simulink library "lib_exhaust2"  (Simulink 5.0)
values from neighbouring files (symbols this model uses):
  logFlag = 1    [advSACompMaskInit.m]    (also in advSACompMaskInitR13.m)
undefined symbols (not defined in the file or in its folder): amb_tmp, cyc_mph, ex_cat_co_frac, ex_cat_ext_cp, ex_cat_ext_emisv, ex_cat_ext_init_tmp, ex_cat_ext_mass, ex_cat_ext_sarea, ex_cat_hc_frac, ex_cat_i2p_th_cond, ex_cat_i2x_emisv, ex_cat_i2x_th_cond, ex_cat_int_cp, ex_cat_int_init_tmp, ex_cat_int_mass, ex_cat_int_sarea, ex_cat_lim, ex_cat_m2i_th_cond, ex_cat_m2i_tmp, ex_cat_m2p_emisv, ex_cat_mon_cp, ex_cat_mon_init_tmp, ex_cat_mon_mass, ex_cat_mon_sarea, ex_cat_monf_sarea, ex_cat_moni_sarea, ex_cat_nox_frac, ex_cat_p2x_th_cond, ex_cat_pcm_ecp, ex_cat_pcm_mass, ex_cat_pcm_tmp, ex_cat_pipe_cp, ex_cat_pipe_emisv, ex_cat_pipe_init_tmp, ex_cat_pipe_mass, ex_cat_pipe_sarea, ex_cat_pm_frac, ex_cat_tmp_range, ex_gas_cp, ex_manif_cp, ex_manif_emisv, ex_manif_init_tmp, ex_manif_mass, ex_manif_sarea, ex_ornl_bool, fc_pwr_scale, magnitude
settings Model: LastModifiedBy=mokeefe
settings Model: ModifiedComment=|
  | mokeefe -- Thu Apr 18 08:32:39 2002 -- Version 1.56
  | saving the model:
  | o "without the model browser open"
  | o with only top-level screen visible
  | o with "fit to view" enabled
  | o with "status bar" off and "toolbar" off
  | o with "prompt to update model history with each save" on
settings Model: ModifiedHistory=|
  | mokeefe -- Thu Apr 18 08:32:39 2002 -- Version 1.56
  | saving the model:
  | o "without the model browser open"
  | o with only top-level screen visible
  | o with "fit to view" enabled
  | o with "status bar" off and "toolbar" off
  | o with "prompt to update model history with each save" on
  | 
  | mokeefe -- Thu Apr 18 08:32:39 2002 -- Version 1.56
  | saving the model:
  | o "without the model browser open"
  | o with only top-level screen visible
  | o with "fit to view" enabled
  | o with "status bar" off and "toolbar" off
  | o with "prompt to update model history with each save" on

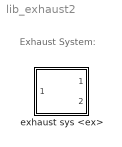
== system lib_exhaust2 ==
  note: Exhaust System:
  exhaust sys <ex> : Subsystem  TreatAsAtomicUnit=on  mask{generalName='ex', logPick=Don't Log, initFileName={}, modCell={}, imgFileName='bdi_ex.jpg', DEBUG=ON}
      mask prompts: generalName "General Name of this Component [char--evaluated]"; logPick "Log Variables to Workspace?"; initFileName "Initialization File(s) [cell array of char]"; modCell "Modification Cell [2 column cell array of param and val]"; imgFileName "Icon image file name [char--evaluated]"
      mask init:
      | % initialization via m-file script
      | advSACompMaskInitR13;
      mask StyleString: edit,popup(Don't Log|Log),edit,edit,edit,popup(ON|OFF)
      mask Display: image(imread(imgFileName))

== system lib_exhaust2/exhaust sys <ex> ==
  EO emis info : Inport
  Exhaust System Model and Interface : Subsystem
  tailpipe emis (g/s) : Outport  OutputWhenDisabled=reset  InitialOutput=0
  cat tmp (C) : Outport  Port=2  OutputWhenDisabled=reset  InitialOutput=0
  tag scope: exReqOut=global, exSensors=global
  wires:
  EO emis info/1 -> Exhaust System Model and Interface/1(EO emis info), [exReqOut]
  Exhaust System Model and Interface/1(tailpipe emis (g/s)) -> tailpipe emis (g/s)/1
  Exhaust System Model and Interface/2(cat tmp (C)) -> cat tmp (C)/1
  [exControl] -> Exhaust System Model and Interface/2(controls)
  Exhaust System Model and Interface/3(sensors) -> [exSensors]

== system lib_exhaust2/exhaust sys <ex>/Exhaust System Model and Interface ==
  note: Interface
  EO emis info : Inport
  controls : Inport  Port=2
  Bus Creator : BusCreator  Inputs=2
  Demux : Demux  Outputs=2
  Goto Tag Visibility : GotoTagVisibility  GotoTag=fc_on
  Model : Subsystem
  tailpipe emis (g/s) : Outport  OutputWhenDisabled=reset  InitialOutput=0
  cat tmp (C) : Outport  Port=2  OutputWhenDisabled=reset  InitialOutput=0
  sensors : Outport  Port=3  OutputWhenDisabled=reset  InitialOutput=0
  tag scope: fc_on=scoped
  wires:
  EO emis info/1 -> Model/1(In1)
  Model/1(tailpipe emis (g/s)) -> tailpipe emis (g/s)/1
  Model/2(cat tmp (C)) -> cat tmp (C)/1
  Bus Creator/1 -> sensors/1

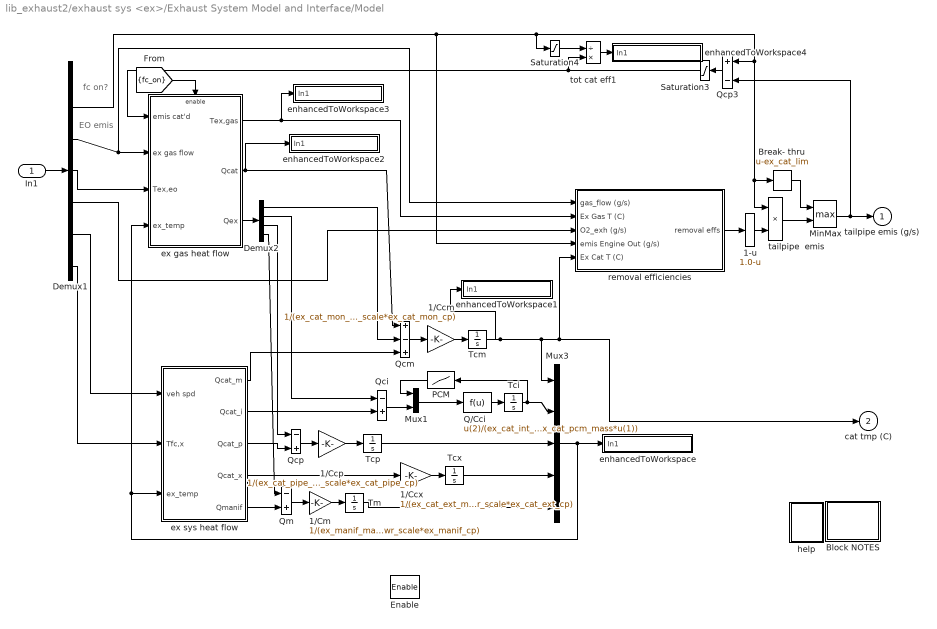
== system lib_exhaust2/exhaust sys <ex>/Exhaust System Model and Interface/Model ==
  note: fc on?
  note: EO emis
  In1 : Inport
  Enable : EnablePort  StatesWhenEnabling=reset
  1-u : MATLABFcn  MATLABFcn=1.0-u
  1/Ccm : Gain  Gain=1/(ex_cat_mon_mass*fc_pwr_scale*ex_cat_mon_cp)  SaturateOnIntegerOverflow=on
  1/Ccp : Gain  Gain=1/(ex_cat_pipe_mass*fc_pwr_scale*ex_cat_pipe_cp)  SaturateOnIntegerOverflow=on
  1/Ccx : Gain  Gain=1/(ex_cat_ext_mass*fc_pwr_scale*ex_cat_ext_cp)  SaturateOnIntegerOverflow=on
  1/Cm : Gain  Gain=1/(ex_manif_mass*fc_pwr_scale*ex_manif_cp)  SaturateOnIntegerOverflow=on
  Block NOTES : Subsystem
      mask Display: disp('Block\nNOTES')
  Break- thru : MATLABFcn  MATLABFcn=u-ex_cat_lim
  Demux1 : Demux  Outputs=[1 4 1 1 1 1 4]
  Demux2 : Demux
  MinMax : MinMax  Function=max  Inputs=2
  Mux1 : Mux  Inputs=2
  Mux3 : Mux  Inputs=5
  PCM : Lookup  Orientation=left  InputValues=ex_cat_pcm_tmp  OutputValues=ex_cat_pcm_ecp  SaturateOnIntegerOverflow=on
  Q/Cci : Fcn  Expr=u(2)/(ex_cat_int_mass*fc_pwr_scale*ex_cat_int_cp+ex_cat_pcm_mass*u(1))
  Qci : Sum  Inputs=-+  SaturateOnIntegerOverflow=on  InputSameDT=on
  Qcm : Sum  Inputs=+-+  SaturateOnIntegerOverflow=on  InputSameDT=on
  Qcp : Sum  Inputs=-+  SaturateOnIntegerOverflow=on  InputSameDT=on
  Qcp3 : Sum  Orientation=left  Inputs=+-  SaturateOnIntegerOverflow=on  InputSameDT=on
  Qm : Sum  Inputs=-+  SaturateOnIntegerOverflow=on  InputSameDT=on
  Saturation3 : Saturate  Orientation=left  UpperLimit=Inf  LowerLimit=0
  Saturation4 : Saturate  UpperLimit=Inf  LowerLimit=eps
  Tci : Integrator  InitialCondition=ex_cat_int_init_tmp
  Tcm : Integrator  InitialCondition=ex_cat_mon_init_tmp
  Tcp : Integrator  InitialCondition=ex_cat_pipe_init_tmp
  Tcx : Integrator  InitialCondition=ex_cat_ext_init_tmp
  Tm : Integrator  InitialCondition=ex_manif_init_tmp
  enhancedToWorkspace : Subsystem  TreatAsAtomicUnit=on  mask(enhancedToWorkspace){generalName=generalName, specificName=tmp, logFlag=logFlag}
      mask prompts: generalName "General Name [char-evaluated]"; specificName "Specific Name [char-literal]"; logFlag "Enable flag (1=on,0=off)"
      mask help: A wrapper for the Simulink "To Workspace" block that allows you to evaluate the name of the variable to log to workspace. This is useful to avoid the double logging errors that occur when you pull in two library models that attempt to log to the same variable.
      mask init:
      | enhancedToWsMaker
      settings: CopyFcn=breakLinkCopyFcn  ParentCloseFcn=breakLinkParCloseFcn
      mask Help:
      | <h2>Enhanced To Workspace Block</h2>
      | <h3>Parameters</h3>
      | <UL>
      | <li><b>General Name:</b> This is the more general name of the variable. Variables are saved to the workspace as <i>generalName_specificName</i>. Note that this is an evaluated variable. If you would like to type in the value directly, it must be surrounded with single quotes. Otherwise you can input the name of a variable containing a char string.</li>
      | <li><b>Specific Name:</b> This is the specific name of the variable. Note that this is input as a char literal (i.e., you don't need quotes).</li>
      | <li><b>Enable Flag:</b> This flag should have the value of 0 or 1. If 0, the variable will not be logged to the workspace. If 1, the variable will be logged. This is done so that variable logging can be turned off to improve speed.</li>
      | </ul>
      | <h3>Overview</h3>
      | <p>The enhanced to workspace block was put together to allow one to dynamically resolve variable names at run time in simulink. This is most powerful when used in conjunction with a masked subsystem to allow multiple instances of that masked subsytem to be used in the same model. The strategy is to set the generalName in the block mask which will allow the block to change the general name for all variable logging on the fly.
      | <h3>Helper Files</h3>
      | <p>Three m-files are required by the enhancedToWorkspace block. These files are located in the &lt; ADVISOR root &gt;/GUI directory :
      | <ul>
      | <li><i>enhancedToWsMaker.m</i> This file runs the mask initialization for the block</li>
      | <li><i>breakLinkCopyFcn.m</i> This file is used by the block callback when the simulink block is copied. It is necessary to break the link to the enhancedToWorkspace similar to the To Workspace block in order for it to be able to configure itself. (Try copying simulink's To Workspace block--it is impossible to make a link)</li>
      | <li><i>breakLinkParCloseFcn.m</i> This file is similar to the breakLinkCopyFcn and is used when a parent system is closed</li>
      | </ul>
      | <hr>
      | 
      | <p>Created 2003-Jan-21, Michael Patrick O'Keefe, NREL</p>
      | 
      | <!--
      | <VARDEF>
      | <H3>var_name</H3>
      | <UL>
      | <LI><B>data type</B> data type here</LI>
      | <LI><B>units</B> units here</LI>
      | <LI><B>vehicle type</B> vehicle type here</LI>
      | <LI><B>description</B> description here</LI>
      | </UL>
      | </VARDEF>
      | -->
      mask Display: disp([generalName,'_',specificName])
  enhancedToWorkspace1 : Subsystem  TreatAsAtomicUnit=on  mask(enhancedToWorkspace){generalName=generalName, specificName=cat_tmp, logFlag=logFlag}
      mask prompts: generalName "General Name [char-evaluated]"; specificName "Specific Name [char-literal]"; logFlag "Enable flag (1=on,0=off)"
      mask help: A wrapper for the Simulink "To Workspace" block that allows you to evaluate the name of the variable to log to workspace. This is useful to avoid the double logging errors that occur when you pull in two library models that attempt to log to the same variable.
      mask init:
      | enhancedToWsMaker
      settings: CopyFcn=breakLinkCopyFcn  ParentCloseFcn=breakLinkParCloseFcn
      mask Help:
      | <h2>Enhanced To Workspace Block</h2>
      | <h3>Parameters</h3>
      | <UL>
      | <li><b>General Name:</b> This is the more general name of the variable. Variables are saved to the workspace as <i>generalName_specificName</i>. Note that this is an evaluated variable. If you would like to type in the value directly, it must be surrounded with single quotes. Otherwise you can input the name of a variable containing a char string.</li>
      | <li><b>Specific Name:</b> This is the specific name of the variable. Note that this is input as a char literal (i.e., you don't need quotes).</li>
      | <li><b>Enable Flag:</b> This flag should have the value of 0 or 1. If 0, the variable will not be logged to the workspace. If 1, the variable will be logged. This is done so that variable logging can be turned off to improve speed.</li>
      | </ul>
      | <h3>Overview</h3>
      | <p>The enhanced to workspace block was put together to allow one to dynamically resolve variable names at run time in simulink. This is most powerful when used in conjunction with a masked subsystem to allow multiple instances of that masked subsytem to be used in the same model. The strategy is to set the generalName in the block mask which will allow the block to change the general name for all variable logging on the fly.
      | <h3>Helper Files</h3>
      | <p>Three m-files are required by the enhancedToWorkspace block. These files are located in the &lt; ADVISOR root &gt;/GUI directory :
      | <ul>
      | <li><i>enhancedToWsMaker.m</i> This file runs the mask initialization for the block</li>
      | <li><i>breakLinkCopyFcn.m</i> This file is used by the block callback when the simulink block is copied. It is necessary to break the link to the enhancedToWorkspace similar to the To Workspace block in order for it to be able to configure itself. (Try copying simulink's To Workspace block--it is impossible to make a link)</li>
      | <li><i>breakLinkParCloseFcn.m</i> This file is similar to the breakLinkCopyFcn and is used when a parent system is closed</li>
      | </ul>
      | <hr>
      | 
      | <p>Created 2003-Jan-21, Michael Patrick O'Keefe, NREL</p>
      | 
      | <!--
      | <VARDEF>
      | <H3>var_name</H3>
      | <UL>
      | <LI><B>data type</B> data type here</LI>
      | <LI><B>units</B> units here</LI>
      | <LI><B>vehicle type</B> vehicle type here</LI>
      | <LI><B>description</B> description here</LI>
      | </UL>
      | </VARDEF>
      | -->
      mask Display: disp([generalName,'_',specificName])
  enhancedToWorkspace2 : Subsystem  TreatAsAtomicUnit=on  mask(enhancedToWorkspace){generalName=generalName, specificName=cat_th_pwr, logFlag=logFlag}
      mask prompts: generalName "General Name [char-evaluated]"; specificName "Specific Name [char-literal]"; logFlag "Enable flag (1=on,0=off)"
      mask help: A wrapper for the Simulink "To Workspace" block that allows you to evaluate the name of the variable to log to workspace. This is useful to avoid the double logging errors that occur when you pull in two library models that attempt to log to the same variable.
      mask init:
      | enhancedToWsMaker
      settings: CopyFcn=breakLinkCopyFcn  ParentCloseFcn=breakLinkParCloseFcn
      mask Help:
      | <h2>Enhanced To Workspace Block</h2>
      | <h3>Parameters</h3>
      | <UL>
      | <li><b>General Name:</b> This is the more general name of the variable. Variables are saved to the workspace as <i>generalName_specificName</i>. Note that this is an evaluated variable. If you would like to type in the value directly, it must be surrounded with single quotes. Otherwise you can input the name of a variable containing a char string.</li>
      | <li><b>Specific Name:</b> This is the specific name of the variable. Note that this is input as a char literal (i.e., you don't need quotes).</li>
      | <li><b>Enable Flag:</b> This flag should have the value of 0 or 1. If 0, the variable will not be logged to the workspace. If 1, the variable will be logged. This is done so that variable logging can be turned off to improve speed.</li>
      | </ul>
      | <h3>Overview</h3>
      | <p>The enhanced to workspace block was put together to allow one to dynamically resolve variable names at run time in simulink. This is most powerful when used in conjunction with a masked subsystem to allow multiple instances of that masked subsytem to be used in the same model. The strategy is to set the generalName in the block mask which will allow the block to change the general name for all variable logging on the fly.
      | <h3>Helper Files</h3>
      | <p>Three m-files are required by the enhancedToWorkspace block. These files are located in the &lt; ADVISOR root &gt;/GUI directory :
      | <ul>
      | <li><i>enhancedToWsMaker.m</i> This file runs the mask initialization for the block</li>
      | <li><i>breakLinkCopyFcn.m</i> This file is used by the block callback when the simulink block is copied. It is necessary to break the link to the enhancedToWorkspace similar to the To Workspace block in order for it to be able to configure itself. (Try copying simulink's To Workspace block--it is impossible to make a link)</li>
      | <li><i>breakLinkParCloseFcn.m</i> This file is similar to the breakLinkCopyFcn and is used when a parent system is closed</li>
      | </ul>
      | <hr>
      | 
      | <p>Created 2003-Jan-21, Michael Patrick O'Keefe, NREL</p>
      | 
      | <!--
      | <VARDEF>
      | <H3>var_name</H3>
      | <UL>
      | <LI><B>data type</B> data type here</LI>
      | <LI><B>units</B> units here</LI>
      | <LI><B>vehicle type</B> vehicle type here</LI>
      | <LI><B>description</B> description here</LI>
      | </UL>
      | </VARDEF>
      | -->
      mask Display: disp([generalName,'_',specificName])
  enhancedToWorkspace3 : Subsystem  TreatAsAtomicUnit=on  mask(enhancedToWorkspace){generalName=generalName, specificName=gas_tmp, logFlag=logFlag}
      mask prompts: generalName "General Name [char-evaluated]"; specificName "Specific Name [char-literal]"; logFlag "Enable flag (1=on,0=off)"
      mask help: A wrapper for the Simulink "To Workspace" block that allows you to evaluate the name of the variable to log to workspace. This is useful to avoid the double logging errors that occur when you pull in two library models that attempt to log to the same variable.
      mask init:
      | enhancedToWsMaker
      settings: CopyFcn=breakLinkCopyFcn  ParentCloseFcn=breakLinkParCloseFcn
      mask Help:
      | <h2>Enhanced To Workspace Block</h2>
      | <h3>Parameters</h3>
      | <UL>
      | <li><b>General Name:</b> This is the more general name of the variable. Variables are saved to the workspace as <i>generalName_specificName</i>. Note that this is an evaluated variable. If you would like to type in the value directly, it must be surrounded with single quotes. Otherwise you can input the name of a variable containing a char string.</li>
      | <li><b>Specific Name:</b> This is the specific name of the variable. Note that this is input as a char literal (i.e., you don't need quotes).</li>
      | <li><b>Enable Flag:</b> This flag should have the value of 0 or 1. If 0, the variable will not be logged to the workspace. If 1, the variable will be logged. This is done so that variable logging can be turned off to improve speed.</li>
      | </ul>
      | <h3>Overview</h3>
      | <p>The enhanced to workspace block was put together to allow one to dynamically resolve variable names at run time in simulink. This is most powerful when used in conjunction with a masked subsystem to allow multiple instances of that masked subsytem to be used in the same model. The strategy is to set the generalName in the block mask which will allow the block to change the general name for all variable logging on the fly.
      | <h3>Helper Files</h3>
      | <p>Three m-files are required by the enhancedToWorkspace block. These files are located in the &lt; ADVISOR root &gt;/GUI directory :
      | <ul>
      | <li><i>enhancedToWsMaker.m</i> This file runs the mask initialization for the block</li>
      | <li><i>breakLinkCopyFcn.m</i> This file is used by the block callback when the simulink block is copied. It is necessary to break the link to the enhancedToWorkspace similar to the To Workspace block in order for it to be able to configure itself. (Try copying simulink's To Workspace block--it is impossible to make a link)</li>
      | <li><i>breakLinkParCloseFcn.m</i> This file is similar to the breakLinkCopyFcn and is used when a parent system is closed</li>
      | </ul>
      | <hr>
      | 
      | <p>Created 2003-Jan-21, Michael Patrick O'Keefe, NREL</p>
      | 
      | <!--
      | <VARDEF>
      | <H3>var_name</H3>
      | <UL>
      | <LI><B>data type</B> data type here</LI>
      | <LI><B>units</B> units here</LI>
      | <LI><B>vehicle type</B> vehicle type here</LI>
      | <LI><B>description</B> description here</LI>
      | </UL>
      | </VARDEF>
      | -->
      mask Display: disp([generalName,'_',specificName])
  enhancedToWorkspace4 : Subsystem  TreatAsAtomicUnit=on  mask(enhancedToWorkspace){generalName=generalName, specificName=cat_eff, logFlag=logFlag}
      mask prompts: generalName "General Name [char-evaluated]"; specificName "Specific Name [char-literal]"; logFlag "Enable flag (1=on,0=off)"
      mask help: A wrapper for the Simulink "To Workspace" block that allows you to evaluate the name of the variable to log to workspace. This is useful to avoid the double logging errors that occur when you pull in two library models that attempt to log to the same variable.
      mask init:
      | enhancedToWsMaker
      settings: CopyFcn=breakLinkCopyFcn  ParentCloseFcn=breakLinkParCloseFcn
      mask Help:
      | <h2>Enhanced To Workspace Block</h2>
      | <h3>Parameters</h3>
      | <UL>
      | <li><b>General Name:</b> This is the more general name of the variable. Variables are saved to the workspace as <i>generalName_specificName</i>. Note that this is an evaluated variable. If you would like to type in the value directly, it must be surrounded with single quotes. Otherwise you can input the name of a variable containing a char string.</li>
      | <li><b>Specific Name:</b> This is the specific name of the variable. Note that this is input as a char literal (i.e., you don't need quotes).</li>
      | <li><b>Enable Flag:</b> This flag should have the value of 0 or 1. If 0, the variable will not be logged to the workspace. If 1, the variable will be logged. This is done so that variable logging can be turned off to improve speed.</li>
      | </ul>
      | <h3>Overview</h3>
      | <p>The enhanced to workspace block was put together to allow one to dynamically resolve variable names at run time in simulink. This is most powerful when used in conjunction with a masked subsystem to allow multiple instances of that masked subsytem to be used in the same model. The strategy is to set the generalName in the block mask which will allow the block to change the general name for all variable logging on the fly.
      | <h3>Helper Files</h3>
      | <p>Three m-files are required by the enhancedToWorkspace block. These files are located in the &lt; ADVISOR root &gt;/GUI directory :
      | <ul>
      | <li><i>enhancedToWsMaker.m</i> This file runs the mask initialization for the block</li>
      | <li><i>breakLinkCopyFcn.m</i> This file is used by the block callback when the simulink block is copied. It is necessary to break the link to the enhancedToWorkspace similar to the To Workspace block in order for it to be able to configure itself. (Try copying simulink's To Workspace block--it is impossible to make a link)</li>
      | <li><i>breakLinkParCloseFcn.m</i> This file is similar to the breakLinkCopyFcn and is used when a parent system is closed</li>
      | </ul>
      | <hr>
      | 
      | <p>Created 2003-Jan-21, Michael Patrick O'Keefe, NREL</p>
      | 
      | <!--
      | <VARDEF>
      | <H3>var_name</H3>
      | <UL>
      | <LI><B>data type</B> data type here</LI>
      | <LI><B>units</B> units here</LI>
      | <LI><B>vehicle type</B> vehicle type here</LI>
      | <LI><B>description</B> description here</LI>
      | </UL>
      | </VARDEF>
      | -->
      mask Display: disp([generalName,'_',specificName])
  ex gas heat flow : Subsystem  TreatAsAtomicUnit=on
  ex sys heat flow : Subsystem
  help : Subsystem
      settings: OpenFcn=web(['file:\\\' which('exhaust.htm')]);
      mask Display: image(imread('doc_man.jpg'))
  removal efficiencies : Subsystem
  tailpipe  emis : Product  SaturateOnIntegerOverflow=on  InputSameDT=on
  tot cat eff1 : Product  Inputs=/*  SaturateOnIntegerOverflow=on  InputSameDT=on
  tailpipe emis (g/s) : Outport  OutputWhenDisabled=reset  InitialOutput=0
  cat tmp (C) : Outport  Port=2  OutputWhenDisabled=reset  InitialOutput=0
  wires:
  ex gas heat flow/3(Qex) -> Demux2/1
  Demux1/4 -> ex gas heat flow/3(Tex,eo)
  1/Ccm/1 -> Tcm/1
  Qcm/1 -> 1/Ccm/1
  ex sys heat flow/1(Qcat_m) -> Qcm/3
  Demux2/1 -> Qcm/2
  ex sys heat flow/4(Qcat_x) -> 1/Ccx/1
  ex sys heat flow/5(Qmanif) -> Qm/2
  ex sys heat flow/2(Qcat_i) -> Qci/2
  1/Ccx/1 -> Tcx/1
  1/Cm/1 -> Tm/1
  Qm/1 -> 1/Cm/1
  Q/Cci/1 -> Tci/1
  Mux1/1 -> Q/Cci/1
  PCM/1 -> Mux1/1
  Qci/1 -> Mux1/2
  Tci/1 -> PCM/1, Mux3/2
  ex sys heat flow/3(Qcat_p) -> Qcp/2
  Demux2/2 -> Qci/1
  Demux2/4 -> Qm/1
  Demux2/3 -> Qcp/1
  Tcx/1 -> Mux3/4
  Tcp/1 -> Mux3/3
  Tm/1 -> Mux3/5
  Mux3/1 -> ex gas heat flow/4(ex_temp), ex sys heat flow/3(ex_temp), enhancedToWorkspace/1(In1)
  Tcm/1 -> Mux3/1, cat tmp (C)/1, removal efficiencies/5(Ex Cat T (C)), enhancedToWorkspace1/1(In1)
  Qcp/1 -> 1/Ccp/1
  1/Ccp/1 -> Tcp/1
  ex gas heat flow/2(Qcat) -> Qcm/1, enhancedToWorkspace2/1(In1)
  Break- thru/1 -> MinMax/1
  tailpipe  emis/1 -> MinMax/2
  1-u/1 -> tailpipe  emis/2
  MinMax/1 -> tailpipe emis (g/s)/1, Qcp3/2
  removal efficiencies/1(removal effs) -> 1-u/1
  Qcp3/1 -> Saturation3/1
  Saturation3/1 -> ex gas heat flow/1(emis cat'd), tot cat eff1/2
  Saturation4/1 -> tot cat eff1/1
  tot cat eff1/1 -> enhancedToWorkspace4/1(In1)
  ex gas heat flow/1(Tex,gas) -> removal efficiencies/2(Ex Gas T (C)), enhancedToWorkspace3/1(In1)
  Demux1/3 -> ex gas heat flow/2(ex gas flow), removal efficiencies/1(gas_flow (g/s))
  Demux1/2 -> Saturation4/1, tailpipe  emis/1, Break- thru/1, Qcp3/1, removal efficiencies/4(emis Engine Out (g/s))
  Demux1/6 -> ex sys heat flow/1(veh spd)
  Demux1/7 -> ex sys heat flow/2(Tfc,x)
  Demux1/5 -> removal efficiencies/3(O2_exh (g/s))
  In1/1 -> Demux1/1
  [fc_on] -> ex gas heat flow/Enable

== system lib_exhaust2/exhaust sys <ex>/Exhaust System Model and Interface/Model/Block NOTES ==
  note: This block models the exhaust system of an internal combustion engine (ICE).  Emphasis is on the catalytic converter
      | aftertreatment of emissions.  Since converter performance is tied to operating temperature, the temperature and heat
      | flows of the exhaust gas, converter, and engine manifold/downpipe are predicted.

== system lib_exhaust2/exhaust sys <ex>/Exhaust System Model and Interface/Model/enhancedToWorkspace ==
  In1 : Inport
  Terminator : Terminator
  wires:
  In1/1 -> Terminator/1

== system lib_exhaust2/exhaust sys <ex>/Exhaust System Model and Interface/Model/enhancedToWorkspace1 ==
  In1 : Inport
  Terminator : Terminator
  wires:
  In1/1 -> Terminator/1

== system lib_exhaust2/exhaust sys <ex>/Exhaust System Model and Interface/Model/enhancedToWorkspace2 ==
  In1 : Inport
  Terminator : Terminator
  wires:
  In1/1 -> Terminator/1

== system lib_exhaust2/exhaust sys <ex>/Exhaust System Model and Interface/Model/enhancedToWorkspace3 ==
  In1 : Inport
  Terminator : Terminator
  wires:
  In1/1 -> Terminator/1

== system lib_exhaust2/exhaust sys <ex>/Exhaust System Model and Interface/Model/enhancedToWorkspace4 ==
  In1 : Inport
  Terminator : Terminator
  wires:
  In1/1 -> Terminator/1

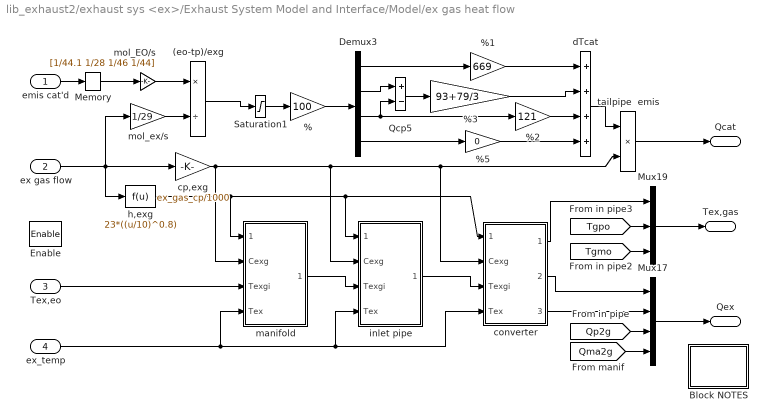
== system lib_exhaust2/exhaust sys <ex>/Exhaust System Model and Interface/Model/ex gas heat flow ==
  emis cat'd : Inport
  ex gas flow : Inport  Port=2
  Tex,eo : Inport  Port=3
  ex_temp : Inport  Port=4
  Enable : EnablePort  StatesWhenEnabling=reset
  % : Gain  Gain=100  SaturateOnIntegerOverflow=on
  %1 : Gain  Gain=669  SaturateOnIntegerOverflow=on
  %2 : Gain  Gain=121  SaturateOnIntegerOverflow=on
  %3 : Gain  Gain=93+79/3  SaturateOnIntegerOverflow=on
  %5 : Gain  Gain=0  SaturateOnIntegerOverflow=on
  (eo-tp)/exg : Product  Inputs=*/  SaturateOnIntegerOverflow=on  InputSameDT=on
  Block NOTES : Subsystem
      mask Display: disp('Block\nNOTES')
  Demux3 : Demux
  Memory : Memory  X0=[0 0 0 0]
  Mux17 : Mux
  Mux19 : Mux  Inputs=3
  Qcp5 : Sum  Inputs=+-  SaturateOnIntegerOverflow=on  InputSameDT=on
  Saturation1 : Saturate  UpperLimit=1  LowerLimit=0
  converter : Subsystem
  cp,exg : Gain  Gain=ex_gas_cp/1000  SaturateOnIntegerOverflow=on
  dTcat : Sum  Inputs=++++  SaturateOnIntegerOverflow=on  InputSameDT=on
  h,exg : Fcn  Expr=23*((u/10)^0.8)
  inlet pipe : Subsystem
  "manifold " : Subsystem
  mol_EO/s : Gain  Gain=[1/44.1 1/28 1/46 1/44]  SaturateOnIntegerOverflow=on
  mol_ex/s : Gain  Gain=1/29  SaturateOnIntegerOverflow=on
  tailpipe  emis : Product  SaturateOnIntegerOverflow=on  InputSameDT=on
  Tex,gas : Outport  OutputWhenDisabled=reset  InitialOutput=amb_tmp
  Qcat : Outport  Port=2  OutputWhenDisabled=reset  InitialOutput=0
  Qex : Outport  Port=3  OutputWhenDisabled=reset  InitialOutput=0
  wires:
  %/1 -> Demux3/1
  h,exg/1 -> "manifold "/1(h,exg), converter/1(h,exg), inlet pipe/1(h,exg)
  cp,exg/1 -> "manifold "/2(Cexg), converter/2(Cexg), tailpipe  emis/2, inlet pipe/2(Cexg)
  ex_temp/1 -> "manifold "/4(Tex), converter/4(Tex), inlet pipe/4(Tex)
  Tex,eo/1 -> "manifold "/3(Texgi)
  (eo-tp)/exg/1 -> Saturation1/1
  mol_EO/s/1 -> (eo-tp)/exg/1
  mol_ex/s/1 -> (eo-tp)/exg/2
  Saturation1/1 -> %/1
  Demux3/4 -> %5/1
  Qcp5/1 -> %3/1
  Demux3/1 -> %1/1
  Demux3/3 -> %2/1, Qcp5/2
  Demux3/2 -> Qcp5/1
  inlet pipe/1(Texgo) -> converter/3(Texgi)
  %5/1 -> dTcat/4
  [Qma2g] -> Mux17/4
  [Qp2g] -> Mux17/3
  converter/3(Qci2g) -> Mux17/2
  converter/2(Qcm2g) -> Mux17/1
  converter/1(Texgo) -> Mux19/1
  [Tgpo] -> Mux19/2
  [Tgmo] -> Mux19/3
  Mux17/1 -> Qex/1
  Mux19/1 -> Tex,gas/1
  tailpipe  emis/1 -> Qcat/1
  dTcat/1 -> tailpipe  emis/1
  %1/1 -> dTcat/1
  %3/1 -> dTcat/2
  %2/1 -> dTcat/3
  "manifold "/1(Texgo) -> inlet pipe/3(Texgi)
  ex gas flow/1 -> mol_ex/s/1, h,exg/1, cp,exg/1
  emis cat'd/1 -> Memory/1
  Memory/1 -> mol_EO/s/1

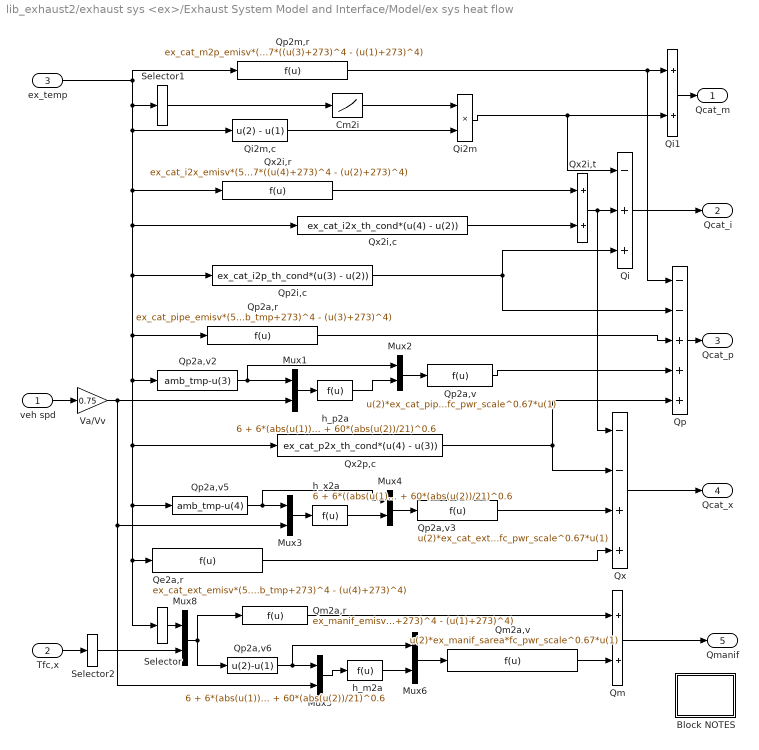
== system lib_exhaust2/exhaust sys <ex>/Exhaust System Model and Interface/Model/ex sys heat flow ==
  veh spd : Inport
  Tfc,x : Inport  Port=2
  ex_temp : Inport  Port=3
  Block NOTES : Subsystem
      mask Display: disp('Block\nNOTES')
  Cm2i : Lookup  InputValues=ex_cat_m2i_tmp  OutputValues=ex_cat_m2i_th_cond  SaturateOnIntegerOverflow=on
  Mux{1..6,8} (7 alike) : Mux  Inputs=2
  Qe2a,r : Fcn  Expr=ex_cat_ext_emisv*(5.67e-8)*ex_cat_ext_sarea*fc_pwr_scale^0.67*((amb_tmp+273)^4 - (u(4)+273)^4)
  Qi : Sum  Inputs=-++  SaturateOnIntegerOverflow=on  InputSameDT=on
  Qi1 : Sum  SaturateOnIntegerOverflow=on  InputSameDT=on
  Qi2m : Product  SaturateOnIntegerOverflow=on  InputSameDT=on
  Qi2m,c : Fcn  Expr=u(2) - u(1)
  Qm : Sum  SaturateOnIntegerOverflow=on  InputSameDT=on
  Qm2a,r : Fcn  Expr=ex_manif_emisv*(5.67e-8)*ex_manif_sarea*fc_pwr_scale^0.67*((u(2)+273)^4 - (u(1)+273)^4)
  Qm2a,v : Fcn  Expr=u(2)*ex_manif_sarea*fc_pwr_scale^0.67*u(1)
  Qp : Sum  Inputs=--+++  SaturateOnIntegerOverflow=on  InputSameDT=on
  Qp2a,r : Fcn  Expr=ex_cat_pipe_emisv*(5.67e-8)*ex_cat_pipe_sarea*fc_pwr_scale^0.67*((amb_tmp+273)^4 - (u(3)+273)^4)
  Qp2a,v : Fcn  Expr=u(2)*ex_cat_pipe_sarea*fc_pwr_scale^0.67*u(1)
  Qp2a,v2 : Fcn  Expr=amb_tmp-u(3)
  Qp2a,v3 : Fcn  Expr=u(2)*ex_cat_ext_sarea*fc_pwr_scale^0.67*u(1)
  Qp2a,v5 : Fcn  Expr=amb_tmp-u(4)
  Qp2a,v6 : Fcn  Expr=u(2)-u(1)
  Qp2i,c : Fcn  Expr=ex_cat_i2p_th_cond*(u(3) - u(2))
  Qp2m,r : Fcn  Expr=ex_cat_m2p_emisv*(5.67e-8)*ex_cat_monf_sarea*fc_pwr_scale^0.67*((u(3)+273)^4 - (u(1)+273)^4)
  Qx : Sum  Inputs=--++  SaturateOnIntegerOverflow=on  InputSameDT=on
  Qx2i,c : Fcn  Expr=ex_cat_i2x_th_cond*(u(4) - u(2))
  Qx2i,r : Fcn  Expr=ex_cat_i2x_emisv*(5.67e-8)*ex_cat_int_sarea*fc_pwr_scale^0.67*((u(4)+273)^4 - (u(2)+273)^4)
  Qx2i,t : Sum  SaturateOnIntegerOverflow=on  InputSameDT=on
  Qx2p,c : Fcn  Expr=ex_cat_p2x_th_cond*(u(4) - u(3))
  Selector : Selector  Elements=5  InputPortWidth=5
  Selector1 : Selector  Elements=[2]  InputPortWidth=5
  Selector2 : Selector  Elements=3  InputPortWidth=4
  Va/Vv : Gain  Gain=0.75  SaturateOnIntegerOverflow=on
  h_m2a : Fcn  Expr=6 + 6*(abs(u(1))/1000)^0.3 + 60*(abs(u(2))/21)^0.6
  h_p2a : Fcn  Expr=6 + 6*(abs(u(1))/1000)^0.3 + 60*(abs(u(2))/21)^0.6
  h_x2a : Fcn  Expr=6 + 6*((abs(u(1))/1000))^0.3 + 60*(abs(u(2))/21)^0.6
  Qcat_m : Outport
  Qcat_i : Outport  Port=2
  Qcat_p : Outport  Port=3
  Qcat_x : Outport  Port=4
  Qmanif : Outport  Port=5
  wires:
  Va/Vv/1 -> Mux1/2, Mux5/2, Mux3/2
  veh spd/1 -> Va/Vv/1
  Selector2/1 -> Mux8/2
  Tfc,x/1 -> Selector2/1
  h_m2a/1 -> Mux6/2
  Mux8/1 -> Qp2a,v6/1, Qm2a,r/1
  Selector/1 -> Mux8/1
  Qp2a,v6/1 -> Mux6/1, Mux5/1
  Mux5/1 -> h_m2a/1
  Mux6/1 -> Qm2a,v/1
  Qm2a,r/1 -> Qm/1
  Qm/1 -> Qmanif/1
  Qm2a,v/1 -> Qm/2
  Qx2p,c/1 -> Qx/2, Qp/5
  h_p2a/1 -> Mux2/2
  Mux2/1 -> Qp2a,v/1
  Qe2a,r/1 -> Qx/4
  h_x2a/1 -> Mux4/2
  Qp2a,v5/1 -> Mux4/1, Mux3/1
  Mux3/1 -> h_x2a/1
  Qp2a,v3/1 -> Qx/3
  Qx2i,t/1 -> Qx/1, Qi/2
  Qx2i,r/1 -> Qx2i,t/1
  Qp2a,v/1 -> Qp/4
  Qp2a,r/1 -> Qp/3
  Qp2m,r/1 -> Qp/1, Qi1/1
  Qp2i,c/1 -> Qp/2, Qi/3
  Cm2i/1 -> Qi2m/1
  Selector1/1 -> Cm2i/1
  Qi2m/1 -> Qi/1, Qi1/2
  Qi2m,c/1 -> Qi2m/2
  Qx2i,c/1 -> Qx2i,t/2
  Qi1/1 -> Qcat_m/1
  Qx/1 -> Qcat_x/1
  Mux4/1 -> Qp2a,v3/1
  Qp2a,v2/1 -> Mux2/1, Mux1/1
  Mux1/1 -> h_p2a/1
  Qp/1 -> Qcat_p/1
  Qi/1 -> Qcat_i/1
  ex_temp/1 -> Selector/1, Qe2a,r/1, Qp2a,v5/1, Qx2p,c/1, Qp2a,v2/1, Qp2a,r/1, Qp2i,c/1, Qi2m,c/1, Selector1/1, Qp2m,r/1, Qx2i,r/1, Qx2i,c/1

== system lib_exhaust2/exhaust sys <ex>/Exhaust System Model and Interface/Model/help ==

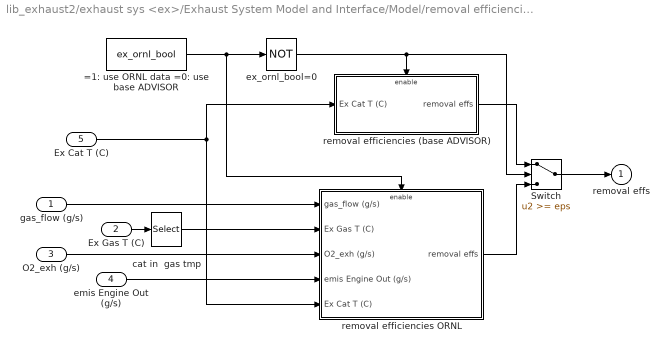
== system lib_exhaust2/exhaust sys <ex>/Exhaust System Model and Interface/Model/removal efficiencies ==
  gas_flow (g/s) : Inport
  Ex Gas T (C) : Inport  Port=2
  O2_exh (g/s) : Inport  Port=3
  emis Engine Out (g/s) : Inport  Port=4
  Ex Cat T (C) : Inport  Port=5
  =1: use ORNL data =0: use base ADVISOR : Constant  Value=ex_ornl_bool
  Switch : Switch  Threshold=eps  SaturateOnIntegerOverflow=on  InputSameDT=on
  cat in  gas tmp : Selector  Elements=2  InputPortWidth=3
  ex_ornl_bool=0 : Logic  Operator=NOT
  removal efficiencies (base ADVISOR) : Subsystem  TreatAsAtomicUnit=on
  removal efficiencies ORNL : Subsystem  TreatAsAtomicUnit=on
  removal effs : Outport  OutputWhenDisabled=reset  InitialOutput=0
  wires:
  ex_ornl_bool=0/1 -> removal efficiencies (base ADVISOR)/Enable, Switch/2
  Ex Cat T (C)/1 -> removal efficiencies (base ADVISOR)/1(Ex Cat T (C)), removal efficiencies ORNL/5(Ex Cat T (C))
  Switch/1 -> removal effs/1
  Ex Gas T (C)/1 -> cat in  gas tmp/1
  cat in  gas tmp/1 -> removal efficiencies ORNL/2(Ex Gas T (C))
  emis Engine Out (g/s)/1 -> removal efficiencies ORNL/4(emis Engine Out (g/s))
  gas_flow (g/s)/1 -> removal efficiencies ORNL/1(gas_flow (g/s))
  O2_exh (g/s)/1 -> removal efficiencies ORNL/3(O2_exh (g/s))
  =1: use ORNL data =0: use base ADVISOR/1 -> ex_ornl_bool=0/1, removal efficiencies ORNL/Enable
  removal efficiencies ORNL/1(removal effs) -> Switch/3
  removal efficiencies (base ADVISOR)/1(removal effs) -> Switch/1

== system lib_exhaust2/exhaust sys <ex>/Exhaust System Model and Interface/Model/ex gas heat flow/Block NOTES ==
  note: EXHAUST GAS HEAT TRANSFER
      | This block models the heat loss from the exhaust gas as it flows from the engine through the manifold,
      | downpipe, and catalytic converter.  Also included is the increase in gas temperature within the converter
      | due to the catalysis of HC, CO, and NOx. The block is conditionally executed only if engine_on=1.

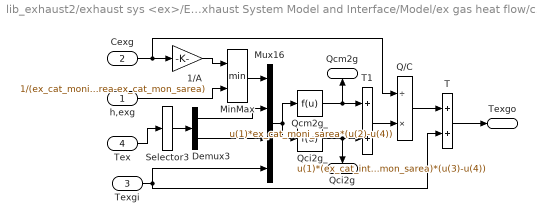
== system lib_exhaust2/exhaust sys <ex>/Exhaust System Model and Interface/Model/ex gas heat flow/converter ==
  h,exg : Inport
  Cexg : Inport  Port=2
  Texgi : Inport  Port=3
  Tex : Inport  Port=4
  " Q/C" : Product  Inputs=/*  SaturateOnIntegerOverflow=on  InputSameDT=on
  1/A : Gain  Gain=1/(ex_cat_moni_sarea+ex_cat_int_sarea-ex_cat_mon_sarea)  SaturateOnIntegerOverflow=on
  Demux3 : Demux  Outputs=2
  MinMax : MinMax  Inputs=2
  Mux16 : Mux
  Qci2g_ : Fcn  Expr=u(1)*(ex_cat_int_sarea - ex_cat_mon_sarea)*(u(3)-u(4))
  Qcm2g_ : Fcn  Expr=u(1)*ex_cat_moni_sarea*(u(2)-u(4))
  Selector3 : Selector  Elements=[ 1 2 ]  InputPortWidth=5
  T : Sum  SaturateOnIntegerOverflow=on  InputSameDT=on
  T1 : Sum  SaturateOnIntegerOverflow=on  InputSameDT=on
  Texgo : Outport  OutputWhenDisabled=reset  InitialOutput=amb_tmp
  Qcm2g : Outport  Orientation=up  Port=2  OutputWhenDisabled=reset  InitialOutput=0
  Qci2g : Outport  Orientation=down  Port=3  OutputWhenDisabled=reset  InitialOutput=0
  wires:
  T/1 -> Texgo/1
  T1/1 -> " Q/C"/2
  " Q/C"/1 -> T/1
  Qcm2g_/1 -> Qcm2g/1, T1/1
  Qci2g_/1 -> Qci2g/1, T1/2
  Mux16/1 -> Qci2g_/1, Qcm2g_/1
  Texgi/1 -> Mux16/4, T/2
  Demux3/2 -> Mux16/3
  Demux3/1 -> Mux16/2
  Selector3/1 -> Demux3/1
  Tex/1 -> Selector3/1
  MinMax/1 -> Mux16/1
  1/A/1 -> MinMax/1
  h,exg/1 -> MinMax/2
  Cexg/1 -> 1/A/1, " Q/C"/1

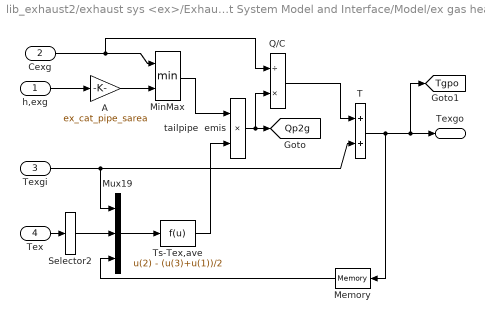
== system lib_exhaust2/exhaust sys <ex>/Exhaust System Model and Interface/Model/ex gas heat flow/inlet pipe ==
  h,exg : Inport
  Cexg : Inport  Port=2
  Texgi : Inport  Port=3
  Tex : Inport  Port=4
  " Q/C" : Product  Inputs=/*  SaturateOnIntegerOverflow=on  InputSameDT=on
  A : Gain  Gain=ex_cat_pipe_sarea  SaturateOnIntegerOverflow=on
  Memory : Memory  Orientation=left  X0=cyc_mph(1,2)*.447
  MinMax : MinMax  Inputs=2
  Mux19 : Mux  Inputs=3
  Selector2 : Selector  Elements=3  InputPortWidth=5
  T : Sum  SaturateOnIntegerOverflow=on  InputSameDT=on
  Ts-Tex,ave : Fcn  Expr=u(2) - (u(3)+u(1))/2
  tailpipe  emis : Product  SaturateOnIntegerOverflow=on  InputSameDT=on
  Texgo : Outport  OutputWhenDisabled=reset  InitialOutput=amb_tmp
  tag scope: Qp2g=global, Tgpo=global
  wires:
  Memory/1 -> Mux19/3
  Selector2/1 -> Mux19/2
  Ts-Tex,ave/1 -> tailpipe  emis/2
  Mux19/1 -> Ts-Tex,ave/1
  Tex/1 -> Selector2/1
  T/1 -> Memory/1, [Tgpo], Texgo/1
  Texgi/1 -> Mux19/1, T/2
  " Q/C"/1 -> T/1
  tailpipe  emis/1 -> [Qp2g], " Q/C"/2
  Cexg/1 -> " Q/C"/1, MinMax/1
  A/1 -> MinMax/2
  MinMax/1 -> tailpipe  emis/1
  h,exg/1 -> A/1

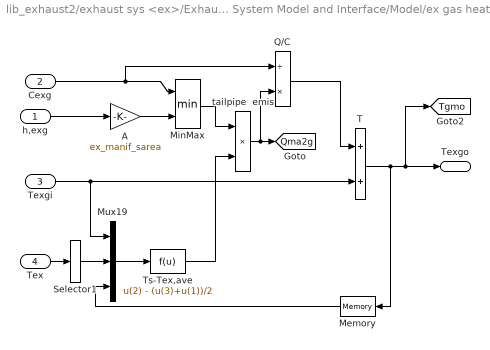
== system lib_exhaust2/exhaust sys <ex>/Exhaust System Model and Interface/Model/ex gas heat flow/manifold  ==
  h,exg : Inport
  Cexg : Inport  Port=2
  Texgi : Inport  Port=3
  Tex : Inport  Port=4
  " Q/C" : Product  Inputs=/*  SaturateOnIntegerOverflow=on  InputSameDT=on
  A : Gain  Gain=ex_manif_sarea  SaturateOnIntegerOverflow=on
  Memory : Memory  Orientation=left  X0=cyc_mph(1,2)*.447
  MinMax : MinMax  Inputs=2
  Mux19 : Mux  Inputs=3
  Selector1 : Selector  Elements=5  InputPortWidth=5
  T : Sum  SaturateOnIntegerOverflow=on  InputSameDT=on
  Ts-Tex,ave : Fcn  Expr=u(2) - (u(3)+u(1))/2
  tailpipe  emis : Product  SaturateOnIntegerOverflow=on  InputSameDT=on
  Texgo : Outport  OutputWhenDisabled=reset  InitialOutput=amb_tmp
  tag scope: Qma2g=global, Tgmo=global
  wires:
  Texgi/1 -> T/2, Mux19/1
  Ts-Tex,ave/1 -> tailpipe  emis/2
  Memory/1 -> Mux19/3
  Mux19/1 -> Ts-Tex,ave/1
  Selector1/1 -> Mux19/2
  Tex/1 -> Selector1/1
  tailpipe  emis/1 -> [Qma2g], " Q/C"/2
  T/1 -> Memory/1, Texgo/1, [Tgmo]
  " Q/C"/1 -> T/1
  Cexg/1 -> " Q/C"/1, MinMax/1
  A/1 -> MinMax/2
  MinMax/1 -> tailpipe  emis/1
  h,exg/1 -> A/1

== system lib_exhaust2/exhaust sys <ex>/Exhaust System Model and Interface/Model/ex sys heat flow/Block NOTES ==
  note: CATALYTIC CONVERTER HEAT LOSS
      | This block models the heat loss from a catalytic converter (conventional or vacuum-insulated).
      | Convection (as a function of vehicle speed), radiation, and conduction effects are included.
      | Converter monolith (m), interior (i), pipe (p), and exterior (x) and engine manifold
      | heat flows are estimated based on the temperatures from the previous iteration.

== system lib_exhaust2/exhaust sys <ex>/Exhaust System Model and Interface/Model/removal efficiencies/removal efficiencies (base ADVISOR) ==
  Ex Cat T (C) : Inport
  Enable : EnablePort  StatesWhenEnabling=reset
  CO temp eff : Lookup  InputValues=ex_cat_tmp_range  OutputValues=ex_cat_co_frac  SaturateOnIntegerOverflow=on
  HC temp eff : Lookup  InputValues=ex_cat_tmp_range  OutputValues=ex_cat_hc_frac  SaturateOnIntegerOverflow=on
  Mux : Mux
  NOx temp eff : Lookup  InputValues=ex_cat_tmp_range  OutputValues=ex_cat_nox_frac  SaturateOnIntegerOverflow=on
  PM temp eff : Lookup  InputValues=ex_cat_tmp_range  OutputValues=ex_cat_pm_frac  SaturateOnIntegerOverflow=on
  removal effs : Outport  OutputWhenDisabled=reset  InitialOutput=0
  wires:
  CO temp eff/1 -> Mux/2
  HC temp eff/1 -> Mux/1
  NOx temp eff/1 -> Mux/3
  PM temp eff/1 -> Mux/4
  Mux/1 -> removal effs/1
  Ex Cat T (C)/1 -> HC temp eff/1, CO temp eff/1, NOx temp eff/1, PM temp eff/1

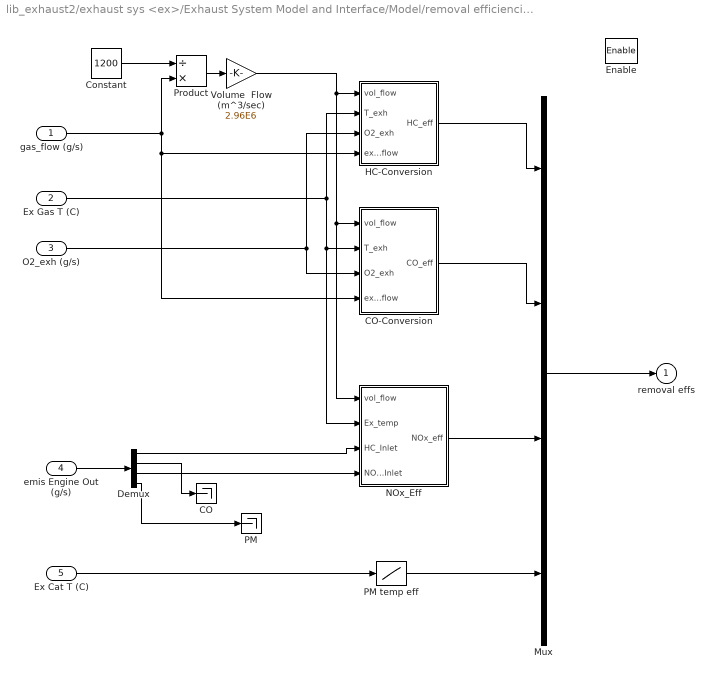
== system lib_exhaust2/exhaust sys <ex>/Exhaust System Model and Interface/Model/removal efficiencies/removal efficiencies ORNL ==
  gas_flow (g/s) : Inport
  Ex Gas T (C) : Inport  Port=2
  O2_exh (g/s) : Inport  Port=3
  emis Engine Out (g/s) : Inport  Port=4
  Ex Cat T (C) : Inport  Port=5
  Enable : EnablePort  StatesWhenEnabling=reset
  CO : Terminator
  CO-Conversion : Subsystem
  Constant : Constant  Value=1200
  Demux : Demux
  HC-Conversion : Subsystem
  Mux : Mux
  NOx_Eff : Subsystem
  PM : Terminator
  PM temp eff : Lookup  InputValues=ex_cat_tmp_range  OutputValues=ex_cat_pm_frac  SaturateOnIntegerOverflow=on
  Product : Product  Inputs=/*  SaturateOnIntegerOverflow=on  InputSameDT=on
  Volume  Flow (m^3/sec) : Gain  Gain=2.96E6  SaturateOnIntegerOverflow=on
  removal effs : Outport  OutputWhenDisabled=reset  InitialOutput=0
  wires:
  Product/1 -> Volume  Flow (m^3/sec)/1
  Constant/1 -> Product/1
  emis Engine Out (g/s)/1 -> Demux/1
  Demux/4 -> PM/1
  Demux/2 -> CO/1
  Demux/3 -> NOx_Eff/4(NOx_Inlet)
  Demux/1 -> NOx_Eff/3(HC_Inlet)
  Volume  Flow (m^3/sec)/1 -> HC-Conversion/1(vol_flow), CO-Conversion/1(vol_flow), NOx_Eff/1(vol_flow)
  Ex Gas T (C)/1 -> HC-Conversion/2(T_exh), CO-Conversion/2(T_exh), NOx_Eff/2(Ex_temp)
  PM temp eff/1 -> Mux/4
  NOx_Eff/1(NOx_eff) -> Mux/3
  HC-Conversion/1(HC_eff) -> Mux/1
  CO-Conversion/1(CO_eff) -> Mux/2
  O2_exh (g/s)/1 -> HC-Conversion/3(O2_exh), CO-Conversion/3(O2_exh)
  Ex Cat T (C)/1 -> PM temp eff/1
  gas_flow (g/s)/1 -> Product/2, HC-Conversion/4(ex_gas_flow), CO-Conversion/4(ex_gas_flow)
  Mux/1 -> removal effs/1

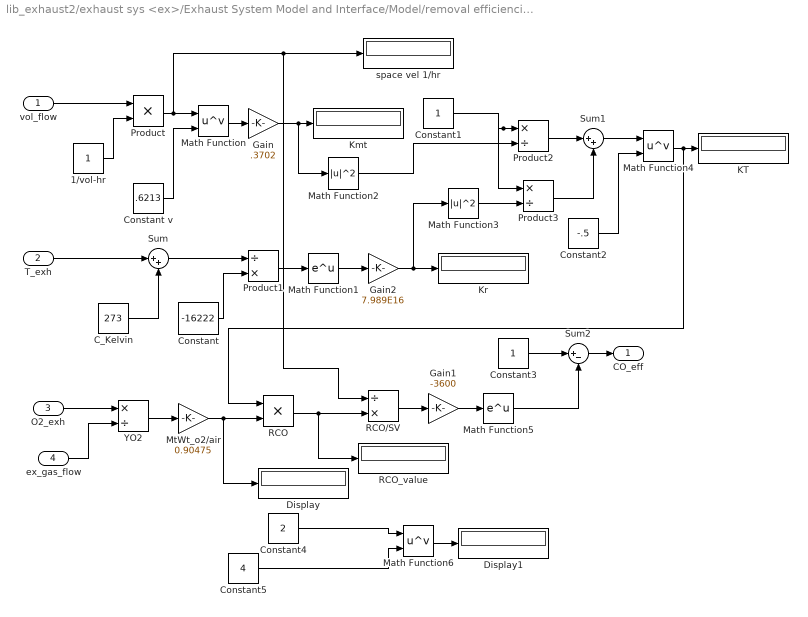
== system lib_exhaust2/exhaust sys <ex>/Exhaust System Model and Interface/Model/removal efficiencies/removal efficiencies ORNL/CO-Conversion ==
  vol_flow : Inport
  T_exh : Inport  Port=2
  O2_exh : Inport  Port=3
  ex_gas_flow : Inport  Port=4
  1/vol-hr : Constant
  C_Kelvin : Constant  Value=273
  Constant : Constant  Value=-16222
  Constant v : Constant  Value=.6213
  Constant1 : Constant
  Constant2 : Constant  Value=-.5
  Constant3 : Constant
  Constant4 : Constant  Value=2
  Constant5 : Constant  Value=4
  Display : Display
  Display1 : Display
  Gain : Gain  Gain=.3702  SaturateOnIntegerOverflow=on
  Gain1 : Gain  Gain=-3600  SaturateOnIntegerOverflow=on
  Gain2 : Gain  Gain=7.989E16  SaturateOnIntegerOverflow=on
  KT : Display
      settings: Format=short_e
  Kmt : Display
      settings: Format=short_e
  Kr : Display
  Math Function : Math  Operator=pow
  Math Function1 : Math
  Math Function2 : Math  Operator=magnitude^2
  Math Function3 : Math  Operator=magnitude^2
  Math Function4 : Math  Operator=pow
  Math Function5 : Math
  Math Function6 : Math  Operator=pow
  MtWt_o2/air : Gain  Gain=0.90475  SaturateOnIntegerOverflow=on
  Product : Product  SaturateOnIntegerOverflow=on  InputSameDT=on
  Product1 : Product  Inputs=/*  SaturateOnIntegerOverflow=on  InputSameDT=on
  Product2 : Product  Inputs=*/  SaturateOnIntegerOverflow=on  InputSameDT=on
  Product3 : Product  Inputs=*/  SaturateOnIntegerOverflow=on  InputSameDT=on
  RCO : Product  SaturateOnIntegerOverflow=on  InputSameDT=on
  RCO/SV : Product  Inputs=/*  SaturateOnIntegerOverflow=on  InputSameDT=on
  RCO_value : Display
  Sum : Sum  Inputs=|++  SaturateOnIntegerOverflow=on  InputSameDT=on
  Sum1 : Sum  Inputs=|++  SaturateOnIntegerOverflow=on  InputSameDT=on
  Sum2 : Sum  Inputs=|+-  SaturateOnIntegerOverflow=on  InputSameDT=on
  YO2 : Product  Inputs=*/  SaturateOnIntegerOverflow=on  InputSameDT=on
  space vel 1/hr : Display
      settings: Format=short_e
  CO_eff : Outport
  wires:
  1/vol-hr/1 -> Product/2
  Constant v/1 -> Math Function/2
  Math Function/1 -> Gain/1
  Product/1 -> Math Function/1, space vel 1/hr/1, RCO/SV/1
  C_Kelvin/1 -> Sum/2
  Constant/1 -> Product1/2
  Sum/1 -> Product1/1
  Math Function1/1 -> Gain2/1
  Gain/1 -> Kmt/1, Math Function2/1
  Gain2/1 -> Kr/1, Math Function3/1
  Constant1/1 -> Product3/1, Product2/1
  Math Function2/1 -> Product2/2
  Math Function3/1 -> Product3/2
  Product2/1 -> Sum1/1
  Product3/1 -> Sum1/2
  Sum1/1 -> Math Function4/1
  Constant2/1 -> Math Function4/2
  Product1/1 -> Math Function1/1
  vol_flow/1 -> Product/1
  T_exh/1 -> Sum/1
  O2_exh/1 -> YO2/1
  ex_gas_flow/1 -> YO2/2
  Math Function4/1 -> KT/1, RCO/1
  RCO/SV/1 -> Gain1/1
  Gain1/1 -> Math Function5/1
  Constant3/1 -> Sum2/1
  Math Function5/1 -> Sum2/2
  Sum2/1 -> CO_eff/1
  RCO/1 -> RCO/SV/2, RCO_value/1
  YO2/1 -> MtWt_o2/air/1
  MtWt_o2/air/1 -> RCO/2, Display/1
  Constant4/1 -> Math Function6/1
  Constant5/1 -> Math Function6/2
  Math Function6/1 -> Display1/1

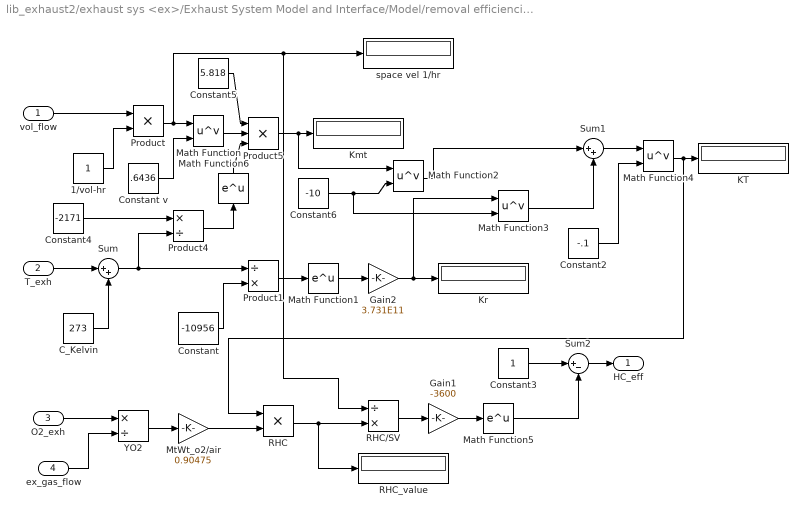
== system lib_exhaust2/exhaust sys <ex>/Exhaust System Model and Interface/Model/removal efficiencies/removal efficiencies ORNL/HC-Conversion ==
  vol_flow : Inport
  T_exh : Inport  Port=2
  O2_exh : Inport  Port=3
  ex_gas_flow : Inport  Port=4
  1/vol-hr : Constant
  C_Kelvin : Constant  Value=273
  Constant : Constant  Value=-10956
  Constant v : Constant  Value=.6436
  Constant2 : Constant  Value=-.1
  Constant3 : Constant
  Constant4 : Constant  Value=-2171
  Constant5 : Constant  Value=5.818
  Constant6 : Constant  Value=-10
  Gain1 : Gain  Gain=-3600  SaturateOnIntegerOverflow=on
  Gain2 : Gain  Gain=3.731E11  SaturateOnIntegerOverflow=on
  KT : Display
      settings: Format=short_e
  Kmt : Display
      settings: Format=short_e
  Kr : Display
  Math Function{,2..4} (4 alike) : Math  Operator=pow
  Math Function1 : Math
  Math Function5 : Math
  Math Function6 : Math  Orientation=up
  MtWt_o2/air : Gain  Gain=0.90475  SaturateOnIntegerOverflow=on
  Product : Product  SaturateOnIntegerOverflow=on  InputSameDT=on
  Product1 : Product  Inputs=/*  SaturateOnIntegerOverflow=on  InputSameDT=on
  Product4 : Product  Inputs=*/  SaturateOnIntegerOverflow=on  InputSameDT=on
  Product5 : Product  Inputs=3  SaturateOnIntegerOverflow=on  InputSameDT=on
  RHC : Product  SaturateOnIntegerOverflow=on  InputSameDT=on
  RHC/SV : Product  Inputs=/*  SaturateOnIntegerOverflow=on  InputSameDT=on
  RHC_value : Display
  Sum : Sum  Inputs=|++  SaturateOnIntegerOverflow=on  InputSameDT=on
  Sum1 : Sum  Inputs=|++  SaturateOnIntegerOverflow=on  InputSameDT=on
  Sum2 : Sum  Inputs=|+-  SaturateOnIntegerOverflow=on  InputSameDT=on
  YO2 : Product  Inputs=*/  SaturateOnIntegerOverflow=on  InputSameDT=on
  space vel 1/hr : Display
      settings: Format=short_e
  HC_eff : Outport
  wires:
  1/vol-hr/1 -> Product/2
  Constant v/1 -> Math Function/2
  Math Function/1 -> Product5/2
  Product/1 -> Math Function/1, space vel 1/hr/1, RHC/SV/1
  C_Kelvin/1 -> Sum/2
  Constant/1 -> Product1/2
  Math Function1/1 -> Gain2/1
  Product5/1 -> Kmt/1, Math Function2/1
  Gain2/1 -> Kr/1, Math Function3/1
  Sum1/1 -> Math Function4/1
  Constant2/1 -> Math Function4/2
  Product1/1 -> Math Function1/1
  vol_flow/1 -> Product/1
  O2_exh/1 -> YO2/1
  ex_gas_flow/1 -> YO2/2
  Math Function4/1 -> KT/1, RHC/1
  RHC/SV/1 -> Gain1/1
  Gain1/1 -> Math Function5/1
  Constant3/1 -> Sum2/1
  Math Function5/1 -> Sum2/2
  Sum2/1 -> HC_eff/1
  YO2/1 -> MtWt_o2/air/1
  MtWt_o2/air/1 -> RHC/2
  RHC/1 -> RHC/SV/2, RHC_value/1
  Constant4/1 -> Product4/1
  Product4/1 -> Math Function6/1
  Constant5/1 -> Product5/1
  Math Function6/1 -> Product5/3
  Constant6/1 -> Math Function2/2, Math Function3/2
  Math Function2/1 -> Sum1/1
  Math Function3/1 -> Sum1/2
  T_exh/1 -> Sum/1
  Sum/1 -> Product1/1, Product4/2

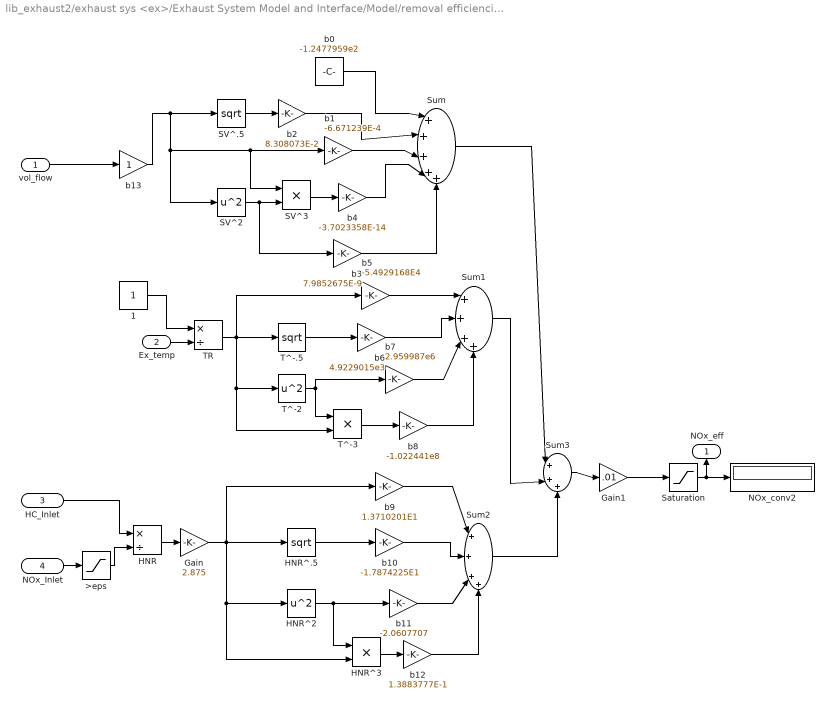
== system lib_exhaust2/exhaust sys <ex>/Exhaust System Model and Interface/Model/removal efficiencies/removal efficiencies ORNL/NOx_Eff ==
  vol_flow : Inport
  Ex_temp : Inport  Port=2
  HC_Inlet : Inport  Port=3
  NOx_Inlet : Inport  Port=4
  1 : Constant
  >eps : Saturate  UpperLimit=inf  LowerLimit=eps
  Gain : Gain  Gain=2.875  SaturateOnIntegerOverflow=on
  Gain1 : Gain  Gain=.01  SaturateOnIntegerOverflow=on
  HNR : Product  Inputs=*/  SaturateOnIntegerOverflow=on  InputSameDT=on
  HNR^.5 : Math  Operator=sqrt
  HNR^2 : Math  Operator=square
  HNR^3 : Product  SaturateOnIntegerOverflow=on  InputSameDT=on
  NOx_conv2 : Display
  SV^.5 : Math  Operator=sqrt
  SV^2 : Math  Operator=square
  SV^3 : Product  SaturateOnIntegerOverflow=on  InputSameDT=on
  Saturation : Saturate  UpperLimit=1.0  LowerLimit=0.0
  Sum : Sum  Inputs=|+++++  SaturateOnIntegerOverflow=on  InputSameDT=on
  Sum1 : Sum  Inputs=|++++  SaturateOnIntegerOverflow=on  InputSameDT=on
  Sum2 : Sum  Inputs=|++++  SaturateOnIntegerOverflow=on  InputSameDT=on
  Sum3 : Sum  Inputs=|+++  SaturateOnIntegerOverflow=on  InputSameDT=on
  TR : Product  Inputs=*/  SaturateOnIntegerOverflow=on  InputSameDT=on
  T^-.5 : Math  Operator=sqrt
  T^-2 : Math  Operator=square
  T^-3 : Product  SaturateOnIntegerOverflow=on  InputSameDT=on
  b0 : Constant  Value=-1.2477959e2
  b1 : Gain  Gain=-6.671239E-4  SaturateOnIntegerOverflow=on
  b10 : Gain  Gain=-1.7874225E1  SaturateOnIntegerOverflow=on
  b11 : Gain  Gain=-2.0607707  SaturateOnIntegerOverflow=on
  b12 : Gain  Gain=1.3883777E-1  SaturateOnIntegerOverflow=on
  b13 : Gain  SaturateOnIntegerOverflow=on
  b2 : Gain  Gain=8.308073E-2  SaturateOnIntegerOverflow=on
  b3 : Gain  Gain=7.9852675E-9  SaturateOnIntegerOverflow=on
  b4 : Gain  Gain=-3.7023358E-14  SaturateOnIntegerOverflow=on
  b5 : Gain  Gain=-5.4929168E4  SaturateOnIntegerOverflow=on
  b6 : Gain  Gain=4.9229015e3  SaturateOnIntegerOverflow=on
  b7 : Gain  Gain=2.959987e6  SaturateOnIntegerOverflow=on
  b8 : Gain  Gain=-1.022441e8  SaturateOnIntegerOverflow=on
  b9 : Gain  Gain=1.3710201E1  SaturateOnIntegerOverflow=on
  NOx_eff : Outport  Orientation=up
  wires:
  vol_flow/1 -> b13/1
  SV^3/1 -> b4/1
  SV^2/1 -> SV^3/2, b3/1
  SV^.5/1 -> b2/1
  b0/1 -> Sum/1
  b2/1 -> Sum/2
  b1/1 -> Sum/3
  b4/1 -> Sum/4
  b3/1 -> Sum/5
  1/1 -> TR/1
  TR/1 -> T^-.5/1, T^-2/1, T^-3/2, b5/1
  T^-3/1 -> b8/1
  T^-2/1 -> T^-3/1, b7/1
  T^-.5/1 -> b6/1
  b5/1 -> Sum1/1
  b6/1 -> Sum1/2
  b7/1 -> Sum1/3
  b8/1 -> Sum1/4
  HNR^3/1 -> b12/1
  HNR^2/1 -> HNR^3/1, b11/1
  HNR^.5/1 -> b10/1
  b9/1 -> Sum2/1
  b10/1 -> Sum2/2
  b11/1 -> Sum2/3
  b12/1 -> Sum2/4
  Sum2/1 -> Sum3/3
  Sum1/1 -> Sum3/2
  Sum/1 -> Sum3/1
  HNR/1 -> Gain/1
  Gain/1 -> HNR^.5/1, b9/1, HNR^3/2, HNR^2/1
  Sum3/1 -> Gain1/1
  Gain1/1 -> Saturation/1
  b13/1 -> SV^.5/1, SV^2/1, b1/1, SV^3/1
  HC_Inlet/1 -> HNR/1
  Ex_temp/1 -> TR/2
  Saturation/1 -> NOx_conv2/1, NOx_eff/1
  NOx_Inlet/1 -> >eps/1
  >eps/1 -> HNR/2
